simulink model "gm_sampleModel2027_3_sub"  (R2023a)
settings: Solver=VariableStepAuto  StartTime=0.0  StopTime=10.0  RelTol=1e-3
libraries: simulink x2, hdlsllib x1
settings Model: Creator=user1  LastModifiedBy=user1
settings OptimizationCC: BlockReduction=off  ConditionallyExecuteInputs=off
settings DebuggingCC: InheritedTsInSrcMsg=none

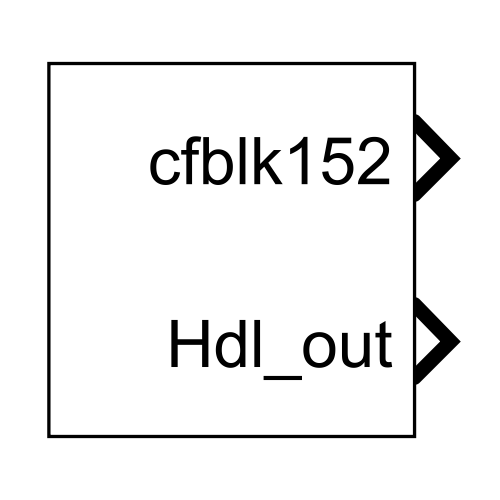
[thumbnail: Simulink's stored preview of the top-level diagram]
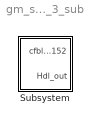
== system gm_sampleModel2027_3_sub ==
  Subsystem : Subsystem

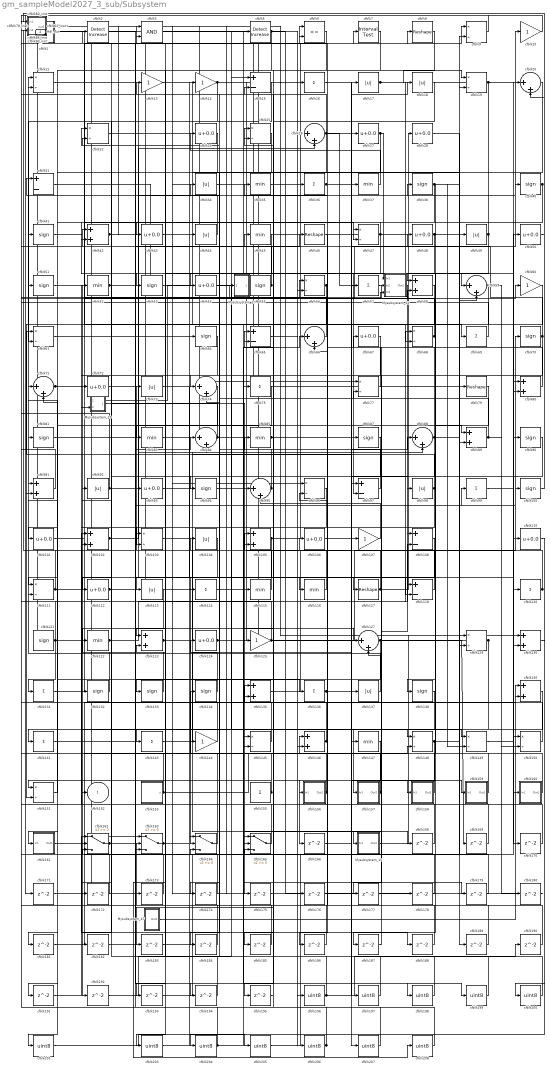
== system gm_sampleModel2027_3_sub/Subsystem ==
  Mysubsystem_15 : Subsystem
  Mysubsystem_19 : Subsystem
  Mysubsystem_29 : Subsystem
  Mysubsystem_47 : Subsystem
  Mysubsystem_52 : Subsystem
  cfblk1 : Subsystem  mask(Detect Rise Positive){vinit=double(0), InputProcessing=Elements as channels (sample based), OutDataTypeStr=uint8}
      mask prompts: vinit "Simulink:masks:InitialCondition_MP"; InputProcessing "Simulink:masks:InputProcessing_MP"; OutDataTypeStr "Simulink:masks:OutputDataType_MP"
      mask help: Simulink:masks:DetectRisePositive_MD
      mask init:
      | InputProcessing = 'Elements as channels (sample based)';
      | OutDataTypeStr = 'uint8';
      | vinit = double(0);
      mask TypeOptions InputProcessing: Simulink:masks:ColumnsAsChannelsFrameBased | Simulink:masks:ElementsAsChannelsSampleBased
      mask TypeOptions OutDataTypeStr: Simulink:masks:uint8 | Simulink:masks:boolean
      mask Display: fprintf('U > 0\n&  NOT\nU/z > 0')
  cfblk{10,13..14,60,107,125,144} (7 alike) : Gain  OutDataTypeStr=uint8
  cfblk{38,40..41,51,53,55,64,70,81,87,90,94,100,121,132..134,138} (18 alike) : Signum
  cfblk{24,27..28,43,48,50,54,67,72,93,101,106,110,112,124} (15 alike) : Bias  Bias=0.0  SaturateOnIntegerOverflow=off
  cfblk{42,58,80,89,91,102,105,123,130,135,140,146} (12 alike) : Sum  OutDataTypeStr=uint8
  cfblk{9,11,19,22,25,47,56,61,68,77,96,103,111,129,145,148..151} (19 alike) : Product  Inputs=*/  OutDataTypeStr=uint8  RndMeth=Zero  SaturateOnIntegerOverflow=on
  cfblk{17..18,34,44,49,73,92,98,104,113,137} (11 alike) : Abs  OutDataTypeStr=uint8  SaturateOnIntegerOverflow=off
  cfblk{15,31,65,97,108,118} (6 alike) : Sum  Inputs=+-  OutDataTypeStr=uint8
  cfblk109_inst : Subsystem
  cfblk{16,36,57,69,75,99,114,120,131,136,141,143} (12 alike) : Sum  Inputs=+  OutDataTypeStr=uint8
  cfblk{35,37,45,52,83,85,115..116,122,147} (10 alike) : MinMax  OutDataTypeStr=uint8
  cfblk{8,46,79,117} (4 alike) : Reshape
  cfblk119_inst : Subsystem
  cfblk126_inst : Subsystem
  cfblk{20,26,59,66,71,74,84,88,95,127} (10 alike) : Sum  Inputs=|++  OutDataTypeStr=uint8
  cfblk12_inst : Subsystem
  cfblk139_inst : Subsystem
  cfblk153 : Subsystem  mask(Counter Free-Running){NumBits=double(16), tsamp=double(-1)}
      mask prompts: NumBits "Simulink:masks:NumberOfBits_MP"; tsamp "Simulink:masks:SampleTime_MP"
      mask help: Simulink:masks:CounterFreeRunning_MD
  cfblk155 : Constant  OutDataTypeStr=uint8  SampleTime=-1
  cfblk156 : Subsystem
  cfblk157 : Subsystem
  cfblk158 : Subsystem
  cfblk159 : Subsystem
  cfblk160 : Subsystem
  cfblk161 : Subsystem
  cfblk{162..165} (4 alike) : Switch  OutDataTypeStr=uint8  SaturateOnIntegerOverflow=off  InputSameDT=off
  cfblk{166,168..195} (29 alike) : Delay  SampleTime=1
  cfblk{196..201,203..208} (12 alike) : DataTypeConversion  OutDataTypeStr=uint8  SaturateOnIntegerOverflow=off  RndMeth=Floor
  cfblk2 : simulink/Logic and Bit Operations/Detect Increase  vinit=0.0  OutDataTypeStr=uint8
      settings: LibrarySourceBlock=|
      | hdlsllib/Logic and Bit
      | Operations/Detect
      | Increase
  cfblk23_inst : Subsystem
  cfblk29_inst : Subsystem
  cfblk3 : Logic  AllPortsSameDT=off  OutDataTypeStr=boolean
  cfblk30_inst : Subsystem
  cfblk33_inst : Subsystem
  cfblk5 : simulink/Logic and Bit Operations/Detect Increase  vinit=0.0  OutDataTypeStr=uint8
      settings: LibrarySourceBlock=|
      | hdlsllib/Logic and Bit
      | Operations/Detect
      | Increase
  cfblk6 : RelationalOperator  Operator=<=  OutDataTypeStr=boolean  InputSameDT=off
  cfblk62_inst : Subsystem
  cfblk7 : hdlsllib/Logic and Bit Operations/Interval Test  IntervalClosedRight=on  uplimit=0.5  IntervalClosedLeft=on  lowlimit=-0.5  OutDataTypeStr=uint8
  cfblk78_inst : Subsystem
  cfblk82_inst : Subsystem
  cfblk86_inst : Subsystem
  cfblk152 : Outport  OutDataTypeStr=uint8  SampleTime=1  VectorParamsAs1DForOutWhenUnconnected=off
  Hdl_out : Outport  Port=2  OutDataTypeStr=uint8  SampleTime=1
  wires:
  Mysubsystem_15/1(Out1) -> cfblk129/1
  Mysubsystem_19/1(Out1) -> Mysubsystem_29/1(In1)
  Mysubsystem_29/1(Out1) -> cfblk175/1
  Mysubsystem_47/1(Out1) -> cfblk140/1
  Mysubsystem_52/1(Out1) -> cfblk183/1
  cfblk1/1(Y) -> cfblk97/2, cfblk47/2, cfblk69/1
  cfblk10/1 -> cfblk171/1
  cfblk100/1 -> cfblk109_inst/1(in1)
  cfblk101/1 -> cfblk9/1
  cfblk102/1 -> cfblk88/2, cfblk26/2
  cfblk103/1 -> Mysubsystem_15/1(In1)
  cfblk104/1 -> cfblk164/2
  cfblk105/1 -> cfblk113/1, cfblk7/1
  cfblk106/1 -> cfblk107/1
  cfblk107/1 -> cfblk95/2
  cfblk108/1 -> cfblk143/1
  cfblk109_inst/1(out1) -> cfblk77/1
  cfblk11/1 -> cfblk170/1
  cfblk110/1 -> cfblk204/1
  cfblk111/1 -> cfblk30_inst/2(in2), Mysubsystem_52/2(In2)
  cfblk112/1 -> cfblk64/1, cfblk56/1
  cfblk113/1 -> cfblk192/1
  cfblk114/1 -> cfblk37/1
  cfblk115/1 -> cfblk11/1
  cfblk116/1 -> cfblk73/1
  cfblk117/1 -> cfblk93/1, cfblk28/1
  cfblk118/1 -> cfblk67/1
  cfblk119_inst/1(out1) -> cfblk130/1
  cfblk12_inst/1(out1) -> cfblk163/1
  cfblk120/1 -> cfblk105/1, cfblk52/1
  cfblk121/1 -> cfblk58/2, cfblk11/2, cfblk131/1
  cfblk122/1 -> cfblk108/2, cfblk68/1
  cfblk123/1 -> cfblk84/2, cfblk168/1
  cfblk124/1 -> cfblk106/1, cfblk5/1
  cfblk125/1 -> cfblk78_inst/1(in1), cfblk70/1
  cfblk126_inst/1(out1) -> cfblk79/1
  cfblk127/1 -> cfblk169/1, cfblk161/1(In1)
  cfblk129/1 -> Hdl_out/1, cfblk157/1(In1)
  cfblk13/1 -> cfblk137/1
  cfblk130/1 -> cfblk200/1
  cfblk131/1 -> cfblk10/1
  cfblk132/1 -> cfblk72/1
  cfblk133/1 -> cfblk102/2
  cfblk134/1 -> cfblk124/1
  cfblk135/1 -> cfblk17/1
  cfblk136/1 -> cfblk18/1, cfblk159/1(In1)
  cfblk137/1 -> cfblk81/1
  cfblk138/1 -> cfblk145/1
  cfblk139_inst/1(out1) -> cfblk115/1, cfblk16/1
  cfblk14/1 -> cfblk61/2, cfblk120/1
  cfblk140/1 -> cfblk201/1
  cfblk141/1 -> cfblk46/1
  cfblk143/1 -> cfblk48/1
  cfblk144/1 -> cfblk29_inst/1(in1)
  cfblk145/1 -> cfblk91/1
  cfblk146/1 -> cfblk66/2, cfblk135/1
  cfblk147/1 -> cfblk195/1
  cfblk148/1 -> cfblk19/2, cfblk166/1
  cfblk149/1 -> cfblk50/1
  cfblk15/1 -> cfblk132/1
  cfblk150/1 -> cfblk42/1
  cfblk151/1 -> cfblk71/1
  cfblk153/1(y) -> cfblk208/1, cfblk148/2, cfblk111/2
  cfblk155/1 -> cfblk23_inst/2(in2), cfblk151/1
  cfblk156/1(Out1) -> cfblk71/2, cfblk122/1
  cfblk157/1(Out1) -> cfblk82_inst/2(in2), cfblk34/1
  cfblk158/1(Out1) -> cfblk6/1
  cfblk159/1(Out1) -> cfblk25/1
  cfblk16/1 -> cfblk98/1
  cfblk160/1(Out1) -> cfblk58/1
  cfblk161/1(Out1) -> cfblk57/1
  cfblk162/1 -> cfblk8/1, cfblk100/1
  cfblk163/1 -> cfblk60/1, cfblk99/1
  cfblk164/1 -> cfblk134/1
  cfblk165/1 -> cfblk92/1
  cfblk166/1 -> cfblk88/1
  cfblk168/1 -> cfblk102/1
  cfblk169/1 -> cfblk123/2
  cfblk17/1 -> cfblk19/1, cfblk148/1
  cfblk170/1 -> cfblk109_inst/2(in2)
  cfblk171/1 -> cfblk146/1
  cfblk172/1 -> cfblk29_inst/2(in2)
  cfblk173/1 -> cfblk162/3
  cfblk174/1 -> cfblk164/3
  cfblk175/1 -> cfblk135/2
  cfblk176/1 -> cfblk96/2
  cfblk177/1 -> cfblk127/2
  cfblk178/1 -> cfblk12_inst/2(in2)
  cfblk179/1 -> cfblk97/1
  cfblk18/1 -> cfblk125/1
  cfblk180/1 -> cfblk1/1(U)
  cfblk181/1 -> cfblk130/2
  cfblk182/1 -> cfblk84/1
  cfblk183/1 -> cfblk89/2
  cfblk184/1 -> cfblk30_inst/1(in1)
  cfblk185/1 -> cfblk163/2
  cfblk186/1 -> cfblk163/3
  cfblk187/1 -> cfblk77/2
  cfblk188/1 -> cfblk119_inst/2(in2)
  cfblk189/1 -> cfblk22/2
  cfblk19/1 -> cfblk150/1, cfblk103/2
  cfblk190/1 -> cfblk6/2
  cfblk191/1 -> cfblk162/1
  cfblk192/1 -> cfblk15/1
  cfblk193/1 -> cfblk80/2
  cfblk194/1 -> cfblk164/1
  cfblk195/1 -> cfblk85/1
  cfblk196/1 -> cfblk27/1, cfblk165/3, cfblk190/1
  cfblk197/1 -> cfblk3/1
  cfblk198/1 -> cfblk3/2
  cfblk199/1 -> cfblk104/1
  cfblk2/1 -> cfblk199/1
  cfblk20/1 -> cfblk114/1
  cfblk200/1 -> cfblk2/1
  cfblk201/1 -> cfblk205/1
  cfblk203/1 -> cfblk140/2
  cfblk204/1 -> cfblk66/1, cfblk23_inst/1(in1)
  cfblk205/1 -> cfblk110/1
  cfblk206/1 -> cfblk62_inst/2(in2), cfblk103/1
  cfblk207/1 -> cfblk65/1
  cfblk208/1 -> cfblk65/2
  cfblk22/1 -> cfblk129/2
  cfblk23_inst/1(out1) -> cfblk96/1
  cfblk24/1 -> cfblk172/1
  cfblk25/1 -> cfblk144/1
  cfblk26/1 -> cfblk86_inst/1(in1), cfblk59/1, cfblk181/1
  cfblk27/1 -> cfblk165/1, Mysubsystem_52/1(In1)
  cfblk28/1 -> cfblk189/1
  cfblk29_inst/1(out1) -> cfblk121/1, cfblk173/1
  cfblk3/1 -> cfblk196/1
  cfblk30_inst/1(out1) -> cfblk49/1, cfblk31/2, cfblk126_inst/1(in1)
  cfblk31/1 -> cfblk55/1
  cfblk33_inst/1(out1) -> cfblk20/1
  cfblk34/1 -> cfblk80/1
  cfblk35/1 -> cfblk15/2
  cfblk36/1 -> cfblk207/1, cfblk118/1
  cfblk37/1 -> cfblk24/1
  cfblk38/1 -> cfblk59/2, cfblk42/2, cfblk149/2, cfblk158/1(In1)
  cfblk40/1 -> cfblk56/2, cfblk141/1
  cfblk41/1 -> cfblk53/1
  cfblk42/1 -> cfblk40/1, cfblk160/1(In1)
  cfblk43/1 -> cfblk75/1
  cfblk44/1 -> cfblk31/1
  cfblk45/1 -> cfblk54/1
  cfblk46/1 -> cfblk156/1(In1)
  cfblk47/1 -> cfblk43/1, cfblk186/1, cfblk185/1
  cfblk48/1 -> cfblk74/2, cfblk123/1
  cfblk49/1 -> cfblk47/1, cfblk187/1
  cfblk5/1 -> cfblk133/1, cfblk68/2, cfblk83/1
  cfblk50/1 -> cfblk20/2
  cfblk51/1 -> cfblk146/2
  cfblk52/1 -> cfblk118/2, cfblk194/1
  cfblk53/1 -> cfblk38/1
  cfblk54/1 -> cfblk149/1
  cfblk55/1 -> cfblk33_inst/2(in2), cfblk126_inst/2(in2)
  cfblk56/1 -> cfblk151/2, cfblk152/1
  cfblk57/1 -> cfblk26/1
  cfblk58/1 -> cfblk91/2
  cfblk59/1 -> cfblk95/1, cfblk180/1
  cfblk6/1 -> cfblk203/1
  cfblk60/1 -> cfblk165/2
  cfblk61/1 -> Mysubsystem_19/1(In1)
  cfblk62_inst/1(out1) -> cfblk44/1
  cfblk64/1 -> cfblk74/1
  cfblk65/1 -> cfblk206/1
  cfblk66/1 -> cfblk86_inst/2(in2)
  cfblk67/1 -> Mysubsystem_29/2(In2)
  cfblk68/1 -> cfblk139_inst/2(in2), cfblk108/1
  cfblk69/1 -> cfblk62_inst/1(in1)
  cfblk7/1 -> cfblk191/1
  cfblk70/1 -> cfblk177/1, cfblk45/1
  cfblk71/1 -> cfblk188/1, cfblk145/2, cfblk111/1, cfblk116/1
  cfblk72/1 -> cfblk89/1
  cfblk73/1 -> cfblk117/1
  cfblk74/1 -> cfblk101/1
  cfblk75/1 -> cfblk184/1
  cfblk77/1 -> cfblk51/1
  cfblk78_inst/1(out1) -> cfblk178/1, cfblk36/1
  cfblk79/1 -> cfblk138/1
  cfblk8/1 -> cfblk105/2
  cfblk80/1 -> cfblk119_inst/1(in1)
  cfblk81/1 -> cfblk136/1
  cfblk82_inst/1(out1) -> cfblk87/1
  cfblk83/1 -> cfblk14/1
  cfblk84/1 -> cfblk198/1, cfblk12_inst/1(in1)
  cfblk85/1 -> cfblk197/1, cfblk147/1
  cfblk86_inst/1(out1) -> cfblk139_inst/1(in1), cfblk176/1
  cfblk87/1 -> cfblk182/1
  cfblk88/1 -> cfblk9/2, cfblk193/1, cfblk35/1
  cfblk89/1 -> cfblk41/1, cfblk150/2
  cfblk9/1 -> cfblk82_inst/1(in1)
  cfblk90/1 -> cfblk112/1
  cfblk91/1 -> cfblk33_inst/1(in1)
  cfblk92/1 -> cfblk78_inst/2(in2), cfblk127/1
  cfblk93/1 -> Mysubsystem_52/3(In3)
  cfblk94/1 -> cfblk179/1
  cfblk95/1 -> cfblk94/1, cfblk13/1
  cfblk96/1 -> cfblk162/2
  cfblk97/1 -> cfblk22/1
  cfblk98/1 -> cfblk61/1, cfblk25/2, cfblk174/1
  cfblk99/1 -> cfblk90/1

== system gm_sampleModel2027_3_sub/Subsystem/Mysubsystem_15 ==
  In1 : Inport  OutDataTypeStr=uint8  PortDimensions=1  SampleTime=1
  cfblk167 : Delay  SampleTime=1
  Out1 : Outport  SampleTime=1
  wires:
  In1/1 -> cfblk167/1
  cfblk167/1 -> Out1/1

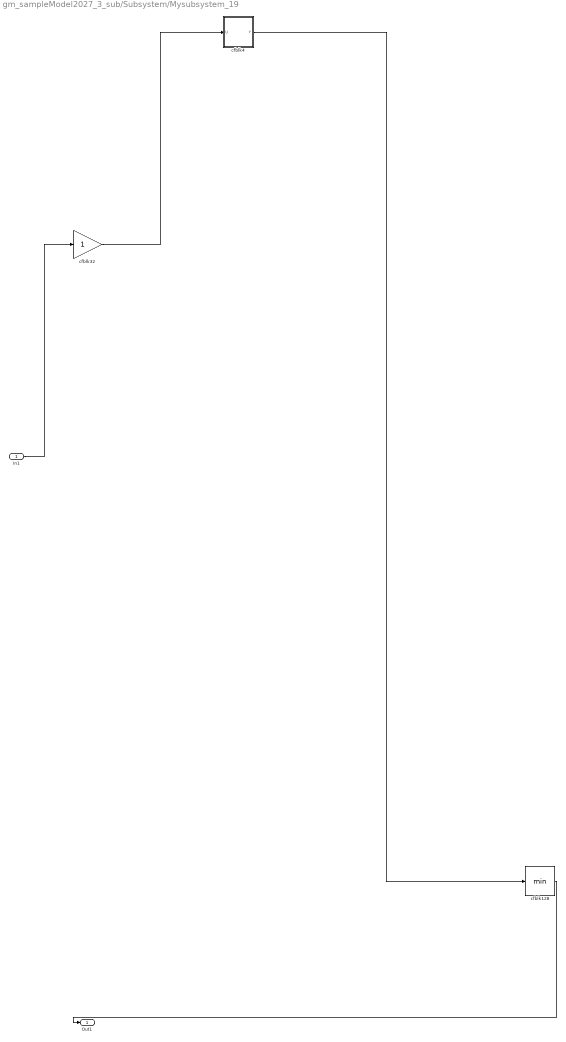
== system gm_sampleModel2027_3_sub/Subsystem/Mysubsystem_19 ==
  In1 : Inport  OutDataTypeStr=uint8  PortDimensions=1  SampleTime=1
  cfblk128 : MinMax
  cfblk32 : Gain
  cfblk4 : Subsystem  mask(Detect Fall Nonpositive){vinit=double(0), InputProcessing=Elements as channels (sample based), OutDataTypeStr=boolean}
      mask prompts: vinit "Simulink:masks:InitialCondition_MP"; InputProcessing "Simulink:masks:InputProcessing_MP"; OutDataTypeStr "Simulink:masks:OutputDataType_MP"
      mask help: Simulink:masks:DetectFallNonpositive_MD
      mask init:
      | InputProcessing = 'Elements as channels (sample based)';
      | OutDataTypeStr = 'boolean';
      | vinit = double(0);
      mask TypeOptions InputProcessing: Simulink:masks:ColumnsAsChannelsFrameBased | Simulink:masks:ElementsAsChannelsSampleBased
      mask TypeOptions OutDataTypeStr: Simulink:masks:uint8 | Simulink:masks:boolean
      mask Display: fprintf('U <= 0\n&  NOT\nU/z <= 0')
  Out1 : Outport  SampleTime=1
  wires:
  In1/1 -> cfblk32/1
  cfblk128/1 -> Out1/1
  cfblk32/1 -> cfblk4/1(U)
  cfblk4/1(Y) -> cfblk128/1

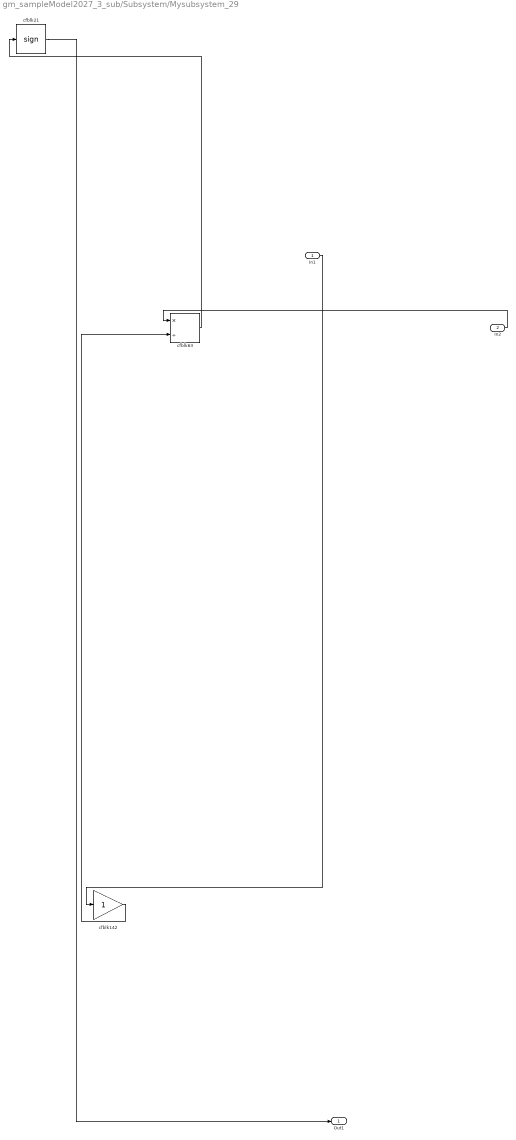
== system gm_sampleModel2027_3_sub/Subsystem/Mysubsystem_29 ==
  In1 : Inport  OutDataTypeStr=boolean  PortDimensions=1  SampleTime=1
  In2 : Inport  Port=2  OutDataTypeStr=uint8  PortDimensions=1  SampleTime=1
  cfblk142 : Gain
  cfblk21 : Signum
  cfblk63 : Product  Inputs=*/  RndMeth=Zero  SaturateOnIntegerOverflow=on
  Out1 : Outport  SampleTime=1
  wires:
  In1/1 -> cfblk142/1
  In2/1 -> cfblk63/1
  cfblk142/1 -> cfblk63/2
  cfblk21/1 -> Out1/1
  cfblk63/1 -> cfblk21/1

== system gm_sampleModel2027_3_sub/Subsystem/Mysubsystem_47 ==
  cfblk154 : Subsystem  mask(Counter Limited){uplimit=double(7), tsamp=double(-1)}
      mask prompts: uplimit "Simulink:masks:UpperLimit_MP"; tsamp "Simulink:masks:SampleTime_MP"
      mask help: Simulink:masks:CounterLimited_MD
      mask init:
      | nbits = double(8);
      | tsamp = double(-1);
      | uplimit = double(7);
  cfblk202 : DataTypeConversion  OutDataTypeStr=uint8  SaturateOnIntegerOverflow=off  RndMeth=Floor
  Out1 : Outport  SampleTime=1
  wires:
  cfblk154/1(y) -> cfblk202/1
  cfblk202/1 -> Out1/1

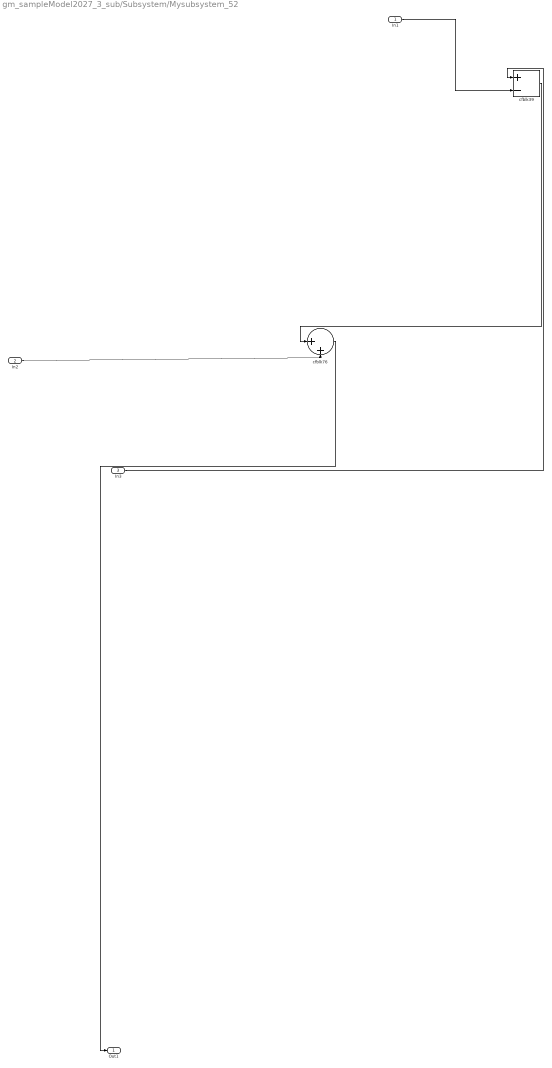
== system gm_sampleModel2027_3_sub/Subsystem/Mysubsystem_52 ==
  In1 : Inport  OutDataTypeStr=uint8  PortDimensions=1  SampleTime=1
  In2 : Inport  Port=2  OutDataTypeStr=uint8  PortDimensions=1  SampleTime=1
  In3 : Inport  Port=3  OutDataTypeStr=uint8  PortDimensions=1  SampleTime=1
  cfblk39 : Sum  Inputs=+-
  cfblk76 : Sum  Inputs=|++
  Out1 : Outport  SampleTime=1
  wires:
  In1/1 -> cfblk39/2
  In2/1 -> cfblk76/2
  In3/1 -> cfblk39/1
  cfblk39/1 -> cfblk76/1
  cfblk76/1 -> Out1/1

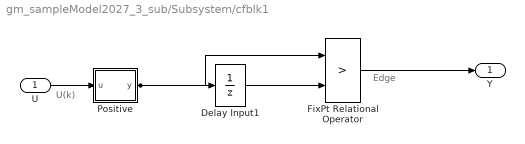
== system gm_sampleModel2027_3_sub/Subsystem/cfblk1 ==
  note: U(k)
  note: Edge
  U : Inport  OutDataTypeStr=uint8  SampleTime=1
  Delay Input1 : UnitDelay  Description=Store in Global RAM  DisableCoverage=on  InitialCondition=vinit  SampleTime=-1  HasFrameUpgradeWarning=on
  FixPt Relational Operator : RelationalOperator  Operator=>  OutDataTypeStr=fixdt(0, 8)  ZeroCross=off  InputSameDT=off
  Positive : Subsystem  mask(Compare To Zero){relop=>, OutDataTypeStr=boolean, ZeroCross=off}
      mask prompts: relop "Simulink:masks:Operator_MP"; OutDataTypeStr "Simulink:masks:OutputDataType_MP"; ZeroCross "Simulink:masks:EnableZerocrossingDetection_MP"
      mask help: Simulink:masks:CompareToZero_MD
      mask init:
      | OutDataTypeStr = 'boolean';
      | ZeroCross = 'off';
      | blkName = 'sampleModel2027_3_sub/Subsystem/cfblk1/Positive';
      | relop = '>';
      | setValue = 'boolean';
      mask TypeOptions relop: == | ~= | < | <= | >= | >
      mask TypeOptions OutDataTypeStr: Simulink:masks:uint8 | Simulink:masks:boolean
      mask Callback ZeroCross: sl('zeroCrossEnable', gcbh);
      mask Display: disp([relop,' 0'])
  Y : Outport  SampleTime=1
  wires:
  U/1 -> Positive/1(u)
  Delay Input1/1 -> FixPt Relational Operator/2
  FixPt Relational Operator/1 -> Y/1
  Positive/1(y) -> FixPt Relational Operator/1, Delay Input1/1

== system gm_sampleModel2027_3_sub/Subsystem/cfblk109_inst ==
  in1 : Inport  OutDataTypeStr=uint8  SampleTime=1
  in2 : Inport  Port=2  OutDataTypeStr=uint8  SampleTime=1
  mul_cfblk109_dotp_mulcomp : Product  Inputs=**  OutDataTypeStr=uint8  SampleTime=1
  out1 : Outport  OutDataTypeStr=uint8  SampleTime=1
  wires:
  in1/1 -> mul_cfblk109_dotp_mulcomp/1
  in2/1 -> mul_cfblk109_dotp_mulcomp/2
  mul_cfblk109_dotp_mulcomp/1 -> out1/1

== system gm_sampleModel2027_3_sub/Subsystem/cfblk119_inst ==
  in1 : Inport  OutDataTypeStr=uint8  SampleTime=1
  in2 : Inport  Port=2  OutDataTypeStr=uint8  SampleTime=1
  mul_cfblk119_dotp_mulcomp : Product  Inputs=**  OutDataTypeStr=uint8  SampleTime=1
  out1 : Outport  OutDataTypeStr=uint8  SampleTime=1
  wires:
  in1/1 -> mul_cfblk119_dotp_mulcomp/1
  in2/1 -> mul_cfblk119_dotp_mulcomp/2
  mul_cfblk119_dotp_mulcomp/1 -> out1/1

== system gm_sampleModel2027_3_sub/Subsystem/cfblk126_inst ==
  in1 : Inport  OutDataTypeStr=uint8  SampleTime=1
  in2 : Inport  Port=2  OutDataTypeStr=uint8  SampleTime=1
  mul_cfblk126_dotp_mulcomp : Product  Inputs=**  OutDataTypeStr=uint8  SampleTime=1
  out1 : Outport  OutDataTypeStr=uint8  SampleTime=1
  wires:
  in1/1 -> mul_cfblk126_dotp_mulcomp/1
  in2/1 -> mul_cfblk126_dotp_mulcomp/2
  mul_cfblk126_dotp_mulcomp/1 -> out1/1

== system gm_sampleModel2027_3_sub/Subsystem/cfblk12_inst ==
  in1 : Inport  OutDataTypeStr=uint8  SampleTime=1
  in2 : Inport  Port=2  OutDataTypeStr=uint8  SampleTime=1
  mul_cfblk12_dotp_mulcomp : Product  Inputs=**  OutDataTypeStr=uint8  SampleTime=1
  out1 : Outport  OutDataTypeStr=uint8  SampleTime=1
  wires:
  in1/1 -> mul_cfblk12_dotp_mulcomp/1
  in2/1 -> mul_cfblk12_dotp_mulcomp/2
  mul_cfblk12_dotp_mulcomp/1 -> out1/1

== system gm_sampleModel2027_3_sub/Subsystem/cfblk139_inst ==
  in1 : Inport  OutDataTypeStr=uint8  SampleTime=1
  in2 : Inport  Port=2  OutDataTypeStr=uint8  SampleTime=1
  mul_cfblk139_dotp_mulcomp : Product  Inputs=**  OutDataTypeStr=uint8  SampleTime=1
  out1 : Outport  OutDataTypeStr=uint8  SampleTime=1
  wires:
  in1/1 -> mul_cfblk139_dotp_mulcomp/1
  in2/1 -> mul_cfblk139_dotp_mulcomp/2
  mul_cfblk139_dotp_mulcomp/1 -> out1/1

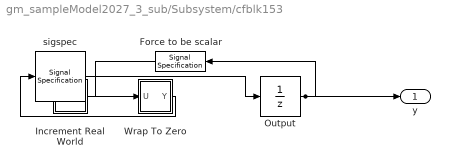
== system gm_sampleModel2027_3_sub/Subsystem/cfblk153 ==
  Force to be scalar : SignalSpecification  DisableCoverage=on  Dimensions=1
  Increment Real World : Subsystem  mask(Real World Value Increment){}
      mask help: Simulink:masks:RealWorldValueIncrement_MD
      mask Display: disp('V++')
  Output : UnitDelay  InitialCondition=0.0  SampleTime=tsamp  HasFrameUpgradeWarning=on
  Wrap To Zero : Subsystem  mask(Wrap To Zero){Threshold=double(65535)}
      mask prompts: Threshold "Simulink:masks:Threshold_MP"
      mask help: Simulink:masks:WrapToZero_MD
  sigspec : SignalSpecification  OutDataTypeStr=uint16  Dimensions=1
  y : Outport  SampleTime=1
  wires:
  Force to be scalar/1 -> Increment Real World/1(u)
  Increment Real World/1(y) -> Wrap To Zero/1(U)
  Output/1 -> Force to be scalar/1, y/1
  Wrap To Zero/1(Y) -> sigspec/1
  sigspec/1 -> Output/1

== system gm_sampleModel2027_3_sub/Subsystem/cfblk156 ==
  In1 : Inport  OutDataTypeStr=uint8  PortDimensions=1  SampleTime=1
  Out1 : Outport  SampleTime=1
  wires:
  In1/1 -> Out1/1

== system gm_sampleModel2027_3_sub/Subsystem/cfblk157 ==
  In1 : Inport  OutDataTypeStr=uint8  PortDimensions=1  SampleTime=1
  Out1 : Outport  SampleTime=1
  wires:
  In1/1 -> Out1/1

== system gm_sampleModel2027_3_sub/Subsystem/cfblk158 ==
  In1 : Inport  OutDataTypeStr=uint8  PortDimensions=1  SampleTime=1
  Out1 : Outport  SampleTime=1
  wires:
  In1/1 -> Out1/1

== system gm_sampleModel2027_3_sub/Subsystem/cfblk159 ==
  In1 : Inport  OutDataTypeStr=uint8  PortDimensions=1  SampleTime=1
  Out1 : Outport  SampleTime=1
  wires:
  In1/1 -> Out1/1

== system gm_sampleModel2027_3_sub/Subsystem/cfblk160 ==
  In1 : Inport  OutDataTypeStr=uint8  PortDimensions=1  SampleTime=1
  Out1 : Outport  SampleTime=1
  wires:
  In1/1 -> Out1/1

== system gm_sampleModel2027_3_sub/Subsystem/cfblk161 ==
  In1 : Inport  OutDataTypeStr=uint8  PortDimensions=1  SampleTime=1
  Out1 : Outport  SampleTime=1
  wires:
  In1/1 -> Out1/1

== system gm_sampleModel2027_3_sub/Subsystem/cfblk23_inst ==
  in1 : Inport  OutDataTypeStr=uint8  SampleTime=1
  in2 : Inport  Port=2  OutDataTypeStr=uint8  SampleTime=1
  mul_cfblk23_dotp_mulcomp : Product  Inputs=**  OutDataTypeStr=uint8  SampleTime=1
  out1 : Outport  OutDataTypeStr=uint8  SampleTime=1
  wires:
  in1/1 -> mul_cfblk23_dotp_mulcomp/1
  in2/1 -> mul_cfblk23_dotp_mulcomp/2
  mul_cfblk23_dotp_mulcomp/1 -> out1/1

== system gm_sampleModel2027_3_sub/Subsystem/cfblk29_inst ==
  in1 : Inport  OutDataTypeStr=uint8  SampleTime=1
  in2 : Inport  Port=2  OutDataTypeStr=uint8  SampleTime=1
  mul_cfblk29_dotp_mulcomp : Product  Inputs=**  OutDataTypeStr=uint8  SampleTime=1
  out1 : Outport  OutDataTypeStr=uint8  SampleTime=1
  wires:
  in1/1 -> mul_cfblk29_dotp_mulcomp/1
  in2/1 -> mul_cfblk29_dotp_mulcomp/2
  mul_cfblk29_dotp_mulcomp/1 -> out1/1

== system gm_sampleModel2027_3_sub/Subsystem/cfblk30_inst ==
  in1 : Inport  OutDataTypeStr=uint8  SampleTime=1
  in2 : Inport  Port=2  OutDataTypeStr=uint8  SampleTime=1
  mul_cfblk30_dotp_mulcomp : Product  Inputs=**  OutDataTypeStr=uint8  SampleTime=1
  out1 : Outport  OutDataTypeStr=uint8  SampleTime=1
  wires:
  in1/1 -> mul_cfblk30_dotp_mulcomp/1
  in2/1 -> mul_cfblk30_dotp_mulcomp/2
  mul_cfblk30_dotp_mulcomp/1 -> out1/1

== system gm_sampleModel2027_3_sub/Subsystem/cfblk33_inst ==
  in1 : Inport  OutDataTypeStr=uint8  SampleTime=1
  in2 : Inport  Port=2  OutDataTypeStr=uint8  SampleTime=1
  mul_cfblk33_dotp_mulcomp : Product  Inputs=**  OutDataTypeStr=uint8  SampleTime=1
  out1 : Outport  OutDataTypeStr=uint8  SampleTime=1
  wires:
  in1/1 -> mul_cfblk33_dotp_mulcomp/1
  in2/1 -> mul_cfblk33_dotp_mulcomp/2
  mul_cfblk33_dotp_mulcomp/1 -> out1/1

== system gm_sampleModel2027_3_sub/Subsystem/cfblk62_inst ==
  in1 : Inport  OutDataTypeStr=uint8  SampleTime=1
  in2 : Inport  Port=2  OutDataTypeStr=uint8  SampleTime=1
  mul_cfblk62_dotp_mulcomp : Product  Inputs=**  OutDataTypeStr=uint8  SampleTime=1
  out1 : Outport  OutDataTypeStr=uint8  SampleTime=1
  wires:
  in1/1 -> mul_cfblk62_dotp_mulcomp/1
  in2/1 -> mul_cfblk62_dotp_mulcomp/2
  mul_cfblk62_dotp_mulcomp/1 -> out1/1

== system gm_sampleModel2027_3_sub/Subsystem/cfblk78_inst ==
  in1 : Inport  OutDataTypeStr=uint8  SampleTime=1
  in2 : Inport  Port=2  OutDataTypeStr=uint8  SampleTime=1
  mul_cfblk78_dotp_mulcomp : Product  Inputs=**  OutDataTypeStr=uint8  SampleTime=1
  out1 : Outport  OutDataTypeStr=uint8  SampleTime=1
  wires:
  in1/1 -> mul_cfblk78_dotp_mulcomp/1
  in2/1 -> mul_cfblk78_dotp_mulcomp/2
  mul_cfblk78_dotp_mulcomp/1 -> out1/1

== system gm_sampleModel2027_3_sub/Subsystem/cfblk82_inst ==
  in1 : Inport  OutDataTypeStr=uint8  SampleTime=1
  in2 : Inport  Port=2  OutDataTypeStr=uint8  SampleTime=1
  mul_cfblk82_dotp_mulcomp : Product  Inputs=**  OutDataTypeStr=uint8  SampleTime=1
  out1 : Outport  OutDataTypeStr=uint8  SampleTime=1
  wires:
  in1/1 -> mul_cfblk82_dotp_mulcomp/1
  in2/1 -> mul_cfblk82_dotp_mulcomp/2
  mul_cfblk82_dotp_mulcomp/1 -> out1/1

== system gm_sampleModel2027_3_sub/Subsystem/cfblk86_inst ==
  in1 : Inport  OutDataTypeStr=uint8  SampleTime=1
  in2 : Inport  Port=2  OutDataTypeStr=uint8  SampleTime=1
  mul_cfblk86_dotp_mulcomp : Product  Inputs=**  OutDataTypeStr=uint8  SampleTime=1
  out1 : Outport  OutDataTypeStr=uint8  SampleTime=1
  wires:
  in1/1 -> mul_cfblk86_dotp_mulcomp/1
  in2/1 -> mul_cfblk86_dotp_mulcomp/2
  mul_cfblk86_dotp_mulcomp/1 -> out1/1

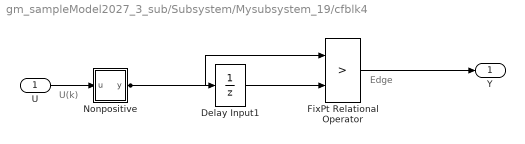
== system gm_sampleModel2027_3_sub/Subsystem/Mysubsystem_19/cfblk4 ==
  note: U(k)
  note: Edge
  U : Inport  OutDataTypeStr=fixdt(0, 16, 7)  SampleTime=1
  Delay Input1 : UnitDelay  Description=Store in Global RAM  DisableCoverage=on  InitialCondition=vinit  SampleTime=-1  HasFrameUpgradeWarning=on
  FixPt Relational Operator : RelationalOperator  Operator=>  OutDataTypeStr=boolean  ZeroCross=off  InputSameDT=off
  Nonpositive : Subsystem  mask(Compare To Zero){relop=<=, OutDataTypeStr=boolean, ZeroCross=off}
      mask prompts: relop "Simulink:masks:Operator_MP"; OutDataTypeStr "Simulink:masks:OutputDataType_MP"; ZeroCross "Simulink:masks:EnableZerocrossingDetection_MP"
      mask help: Simulink:masks:CompareToZero_MD
      mask init:
      | OutDataTypeStr = 'boolean';
      | ZeroCross = 'off';
      | blkName = 'sampleModel2027_3_sub/Subsystem/Mysubsystem_19/cfblk4/Nonpositive';
      | relop = '<=';
      | setValue = 'boolean';
      mask TypeOptions relop: == | ~= | < | <= | >= | >
      mask TypeOptions OutDataTypeStr: Simulink:masks:uint8 | Simulink:masks:boolean
      mask Callback ZeroCross: sl('zeroCrossEnable', gcbh);
      mask Display: disp([relop,' 0'])
  Y : Outport  SampleTime=1
  wires:
  U/1 -> Nonpositive/1(u)
  Delay Input1/1 -> FixPt Relational Operator/2
  FixPt Relational Operator/1 -> Y/1
  Nonpositive/1(y) -> FixPt Relational Operator/1, Delay Input1/1

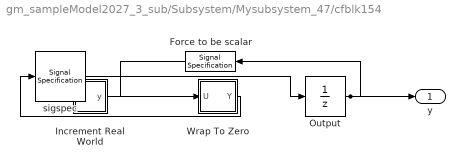
== system gm_sampleModel2027_3_sub/Subsystem/Mysubsystem_47/cfblk154 ==
  Force to be scalar : SignalSpecification  DisableCoverage=on  Dimensions=1
  Increment Real World : Subsystem  mask(Real World Value Increment){}
      mask help: Simulink:masks:RealWorldValueIncrement_MD
      mask Display: disp('V++')
  Output : UnitDelay  InitialCondition=0.0  SampleTime=tsamp  HasFrameUpgradeWarning=on
  Wrap To Zero : Subsystem  mask(Wrap To Zero){Threshold=double(7)}
      mask prompts: Threshold "Simulink:masks:Threshold_MP"
      mask help: Simulink:masks:WrapToZero_MD
  sigspec : SignalSpecification  OutDataTypeStr=uint8  Dimensions=1
  y : Outport  SampleTime=1
  wires:
  Force to be scalar/1 -> Increment Real World/1(u)
  Increment Real World/1(y) -> Wrap To Zero/1(U)
  Output/1 -> Force to be scalar/1, y/1
  Wrap To Zero/1(Y) -> sigspec/1
  sigspec/1 -> Output/1

== system gm_sampleModel2027_3_sub/Subsystem/cfblk1/Positive ==
  u : Inport  OutDataTypeStr=uint8  SampleTime=1
  Compare : RelationalOperator  Operator=>  OutDataTypeStr=boolean  ZeroCross=off
  Constant : Constant  DisableCoverage=on  Value=0  OutDataTypeStr=Inherit: Inherit via back propagation  SampleTime=-1  PreserveConstantTs=on
  y : Outport  SampleTime=1
  wires:
  u/1 -> Compare/1
  Compare/1 -> y/1
  Constant/1 -> Compare/2

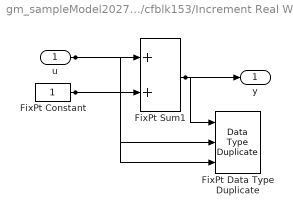
== system gm_sampleModel2027_3_sub/Subsystem/cfblk153/Increment Real World ==
  u : Inport  OutDataTypeStr=uint16  SampleTime=1
  FixPt Constant : Constant  DisableCoverage=on  OutDataTypeStr=Inherit: Inherit via back propagation  SampleTime=-1
  FixPt Data Type Duplicate : DataTypeDuplicate  DisableCoverage=on  NumInputPorts=3
  FixPt Sum1 : Sum  InputSameDT=on  OutDataTypeStr=Inherit: Inherit via back propagation  LockScale=on
  y : Outport  SampleTime=1
  wires:
  u/1 -> FixPt Sum1/1, FixPt Data Type Duplicate/2
  FixPt Constant/1 -> FixPt Sum1/2, FixPt Data Type Duplicate/3
  FixPt Sum1/1 -> FixPt Data Type Duplicate/1, y/1

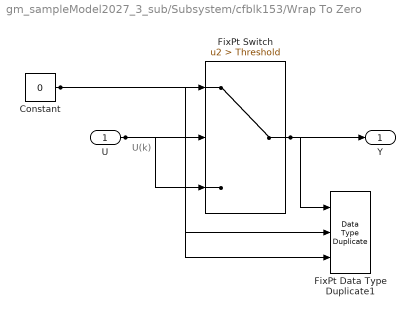
== system gm_sampleModel2027_3_sub/Subsystem/cfblk153/Wrap To Zero ==
  note: U(k)
  U : Inport  OutDataTypeStr=uint16  SampleTime=1
  Constant : Constant  DisableCoverage=on  Value=0  OutDataTypeStr=Inherit: Inherit via back propagation  SampleTime=-1
  FixPt Data Type Duplicate1 : DataTypeDuplicate  DisableCoverage=on  NumInputPorts=3
  FixPt Switch : Switch  Criteria=u2 > Threshold  Threshold=Threshold  OutDataTypeStr=Inherit: Inherit via back propagation  ZeroCross=off  SaturateOnIntegerOverflow=off  InputSameDT=off
  Y : Outport  SampleTime=1
  wires:
  U/1 -> FixPt Switch/3, FixPt Switch/2, FixPt Data Type Duplicate1/2
  Constant/1 -> FixPt Switch/1, FixPt Data Type Duplicate1/3
  FixPt Switch/1 -> FixPt Data Type Duplicate1/1, Y/1

== system gm_sampleModel2027_3_sub/Subsystem/Mysubsystem_19/cfblk4/Nonpositive ==
  u : Inport  OutDataTypeStr=fixdt(0, 16, 7)  SampleTime=1
  Compare : RelationalOperator  Operator=<=  OutDataTypeStr=boolean  ZeroCross=off
  Constant : Constant  DisableCoverage=on  Value=0  OutDataTypeStr=Inherit: Inherit via back propagation  SampleTime=-1  PreserveConstantTs=on
  y : Outport  SampleTime=1
  wires:
  u/1 -> Compare/1
  Compare/1 -> y/1
  Constant/1 -> Compare/2

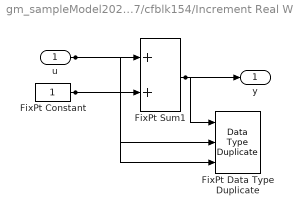
== system gm_sampleModel2027_3_sub/Subsystem/Mysubsystem_47/cfblk154/Increment Real World ==
  u : Inport  OutDataTypeStr=uint8  SampleTime=1
  FixPt Constant : Constant  DisableCoverage=on  OutDataTypeStr=Inherit: Inherit via back propagation  SampleTime=-1
  FixPt Data Type Duplicate : DataTypeDuplicate  DisableCoverage=on  NumInputPorts=3
  FixPt Sum1 : Sum  InputSameDT=on  OutDataTypeStr=Inherit: Inherit via back propagation  LockScale=on
  y : Outport  SampleTime=1
  wires:
  u/1 -> FixPt Sum1/1, FixPt Data Type Duplicate/2
  FixPt Constant/1 -> FixPt Sum1/2, FixPt Data Type Duplicate/3
  FixPt Sum1/1 -> FixPt Data Type Duplicate/1, y/1

== system gm_sampleModel2027_3_sub/Subsystem/Mysubsystem_47/cfblk154/Wrap To Zero ==
  note: U(k)
  U : Inport  OutDataTypeStr=uint8  SampleTime=1
  Constant : Constant  DisableCoverage=on  Value=0  OutDataTypeStr=Inherit: Inherit via back propagation  SampleTime=-1
  FixPt Data Type Duplicate1 : DataTypeDuplicate  DisableCoverage=on  NumInputPorts=3
  FixPt Switch : Switch  Criteria=u2 > Threshold  Threshold=Threshold  OutDataTypeStr=Inherit: Inherit via back propagation  ZeroCross=off  SaturateOnIntegerOverflow=off  InputSameDT=off
  Y : Outport  SampleTime=1
  wires:
  U/1 -> FixPt Switch/3, FixPt Switch/2, FixPt Data Type Duplicate1/2
  Constant/1 -> FixPt Switch/1, FixPt Data Type Duplicate1/3
  FixPt Switch/1 -> FixPt Data Type Duplicate1/1, Y/1
